simulink model "gm_sampleModel1598_5_sub"  (R2023a)
settings: Solver=VariableStepAuto  StartTime=0.0  StopTime=10.0  RelTol=1e-3
libraries: simulink x3
settings Model: Creator=user1  LastModifiedBy=user1
settings OptimizationCC: BlockReduction=off  ConditionallyExecuteInputs=off
settings DebuggingCC: InheritedTsInSrcMsg=none

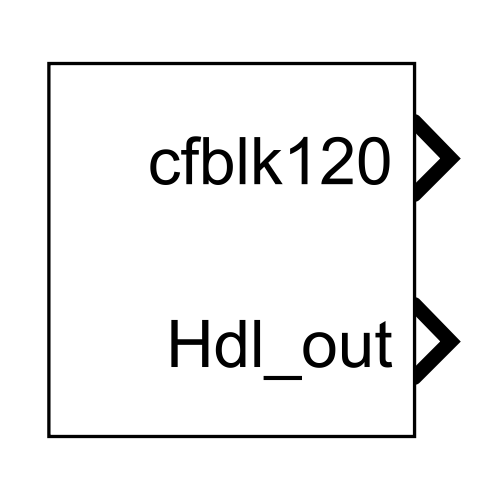
[thumbnail: Simulink's stored preview of the top-level diagram]
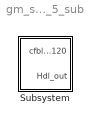
== system gm_sampleModel1598_5_sub ==
  Subsystem : Subsystem

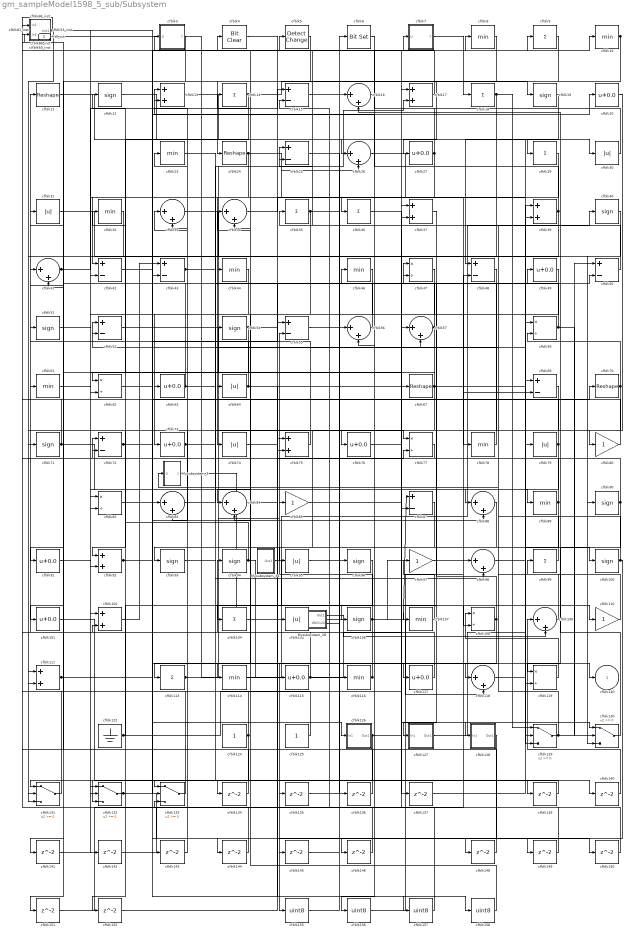
== system gm_sampleModel1598_5_sub/Subsystem ==
  Mysubsystem_28 : Subsystem
  Mysubsystem_3 : Subsystem
  Mysubsystem_34 : Subsystem
  cfblk{8,10,23,32,44,46,61,78,89,107,114,116} (12 alike) : MinMax  OutDataTypeStr=uint8
  cfblk{12,19,40,51,54,71,90,93..94,96,100,106} (12 alike) : Signum
  cfblk{20,27,49,63,73,76,91,101,115,117} (10 alike) : Bias  Bias=0.0  SaturateOnIntegerOverflow=off
  cfblk{13,17,37,39,75,92,102,111} (8 alike) : Sum  OutDataTypeStr=uint8
  cfblk103_inst : Subsystem
  cfblk{9,14,18,29,35..36,99,104,113} (9 alike) : Sum  Inputs=+  OutDataTypeStr=uint8
  cfblk{30..31,64,74,79,95,105} (7 alike) : Abs  OutDataTypeStr=uint8  SaturateOnIntegerOverflow=off
  cfblk{47,59,62,77,82,108,119} (7 alike) : Product  Inputs=*/  OutDataTypeStr=uint8  RndMeth=Zero  SaturateOnIntegerOverflow=on
  cfblk{16,26,33..34,41,56..57,83..84,88,98,109,118} (13 alike) : Sum  Inputs=|++  OutDataTypeStr=uint8
  cfblk{11,24,67,70} (4 alike) : Reshape
  cfblk{80,85,97,110} (4 alike) : Gain  OutDataTypeStr=uint8
  cfblk122 : Ground
  cfblk124 : Constant  OutDataTypeStr=uint8  SampleTime=-1
  cfblk125 : Constant  OutDataTypeStr=uint8  SampleTime=-1
  cfblk126 : Subsystem
  cfblk127 : Subsystem
  cfblk128 : Subsystem
  cfblk{129..133} (5 alike) : Switch  OutDataTypeStr=uint8  SaturateOnIntegerOverflow=off  InputSameDT=off
  cfblk{134..137,139..146,148..152} (17 alike) : Delay  SampleTime=1
  cfblk{15,25,42..43,48,50,52,55,69,72,87} (11 alike) : Sum  Inputs=+-  OutDataTypeStr=uint8
  cfblk{155..158} (4 alike) : DataTypeConversion  OutDataTypeStr=uint8  SaturateOnIntegerOverflow=off  RndMeth=Floor
  cfblk21_inst : Subsystem
  cfblk28_inst : Subsystem
  cfblk3 : Subsystem  mask(Detect Rise Positive){vinit=double(0), InputProcessing=Elements as channels (sample based), OutDataTypeStr=uint8}
      mask prompts: vinit "Simulink:masks:InitialCondition_MP"; InputProcessing "Simulink:masks:InputProcessing_MP"; OutDataTypeStr "Simulink:masks:OutputDataType_MP"
      mask help: Simulink:masks:DetectRisePositive_MD
      mask init:
      | InputProcessing = 'Elements as channels (sample based)';
      | OutDataTypeStr = 'uint8';
      | vinit = double(0);
      mask TypeOptions InputProcessing: Simulink:masks:ColumnsAsChannelsFrameBased | Simulink:masks:ElementsAsChannelsSampleBased
      mask TypeOptions OutDataTypeStr: Simulink:masks:uint8 | Simulink:masks:boolean
      mask Display: fprintf('U > 0\n&  NOT\nU/z > 0')
  cfblk38_inst : Subsystem
  cfblk4 : simulink/Logic and Bit Operations/Bit Clear  iBit=0
      settings: LibrarySourceBlock=|
      | hdlsllib/Logic and Bit
      | Operations/Bit Clear
  cfblk5 : simulink/Logic and Bit Operations/Detect Change  vinit=0  OutDataTypeStr=uint8
      settings: LibrarySourceBlock=|
      | hdlsllib/Logic and Bit
      | Operations/Detect
      | Change
  cfblk53_inst : Subsystem
  cfblk6 : simulink/Logic and Bit Operations/Bit Set  iBit=0
      settings: LibrarySourceBlock=|
      | hdlsllib/Logic and Bit
      | Operations/Bit Set
  cfblk60_inst : Subsystem
  cfblk68_inst : Subsystem
  cfblk7 : Subsystem  mask(Detect Fall Nonpositive){vinit=double(0), InputProcessing=Elements as channels (sample based), OutDataTypeStr=uint8}
      mask prompts: vinit "Simulink:masks:InitialCondition_MP"; InputProcessing "Simulink:masks:InputProcessing_MP"; OutDataTypeStr "Simulink:masks:OutputDataType_MP"
      mask help: Simulink:masks:DetectFallNonpositive_MD
      mask init:
      | InputProcessing = 'Elements as channels (sample based)';
      | OutDataTypeStr = 'uint8';
      | vinit = double(0);
      mask TypeOptions InputProcessing: Simulink:masks:ColumnsAsChannelsFrameBased | Simulink:masks:ElementsAsChannelsSampleBased
      mask TypeOptions OutDataTypeStr: Simulink:masks:uint8 | Simulink:masks:boolean
      mask Display: fprintf('U <= 0\n&  NOT\nU/z <= 0')
  cfblk81_inst : Subsystem
  cfblk86_inst : Subsystem
  cfblk120 : Outport  OutDataTypeStr=uint8  SampleTime=1  VectorParamsAs1DForOutWhenUnconnected=off
  Hdl_out : Outport  Port=2  OutDataTypeStr=uint8  SampleTime=1
  wires:
  Mysubsystem_28/1(Out1) -> cfblk109/2
  Mysubsystem_28/2(cfblk120) -> cfblk120/1
  Mysubsystem_3/1(Out1) -> Mysubsystem_28/1(In1)
  Mysubsystem_34/1(Out1) -> cfblk106/1
  cfblk10/1 -> cfblk56/2, cfblk24/1
  cfblk100/1 -> cfblk148/1, Mysubsystem_3/1(U)
  cfblk101/1 -> cfblk134/1
  cfblk102/1 -> cfblk43/1
  cfblk103_inst/1(out1) -> cfblk38_inst/2(in2)
  cfblk104/1 -> cfblk110/1
  cfblk105/1 -> cfblk98/1
  cfblk106/1 -> cfblk87/1, cfblk55/2, cfblk118/2, cfblk102/2
  cfblk107/1 -> cfblk97/1
  cfblk108/1 -> cfblk155/1, cfblk47/1, cfblk113/1
  cfblk109/1 -> cfblk99/1
  cfblk11/1 -> cfblk29/1
  cfblk110/1 -> cfblk35/1
  cfblk111/1 -> cfblk55/1, cfblk140/1
  cfblk113/1 -> cfblk17/2, cfblk85/1
  cfblk114/1 -> cfblk40/1
  cfblk115/1 -> cfblk87/2, cfblk81_inst/2(in2)
  cfblk116/1 -> cfblk94/1, cfblk11/1, Hdl_out/1
  cfblk117/1 -> cfblk103_inst/1(in1)
  cfblk118/1 -> cfblk79/1
  cfblk119/1 -> cfblk108/1
  cfblk12/1 -> cfblk26/1
  cfblk122/1 -> cfblk57/1, cfblk52/1
  cfblk124/1 -> cfblk53_inst/2(in2), cfblk33/2, cfblk133/1
  cfblk125/1 -> cfblk72/1
  cfblk126/1(Out1) -> cfblk37/1, cfblk132/3
  cfblk127/1(Out1) -> cfblk39/1
  cfblk128/1(Out1) -> cfblk145/1
  cfblk129/1 -> cfblk52/2, cfblk50/1, cfblk61/1
  cfblk13/1 -> cfblk69/1
  cfblk130/1 -> cfblk16/2
  cfblk131/1 -> cfblk60_inst/2(in2)
  cfblk132/1 -> cfblk88/2, cfblk144/1
  cfblk133/1 -> cfblk68_inst/2(in2)
  cfblk134/1 -> cfblk41/1
  cfblk135/1 -> cfblk16/1
  cfblk136/1 -> cfblk68_inst/1(in1)
  cfblk137/1 -> cfblk39/2
  cfblk139/1 -> cfblk131/1
  cfblk14/1 -> cfblk19/1, cfblk62/1
  cfblk140/1 -> cfblk109/1
  cfblk141/1 -> cfblk37/2
  cfblk142/1 -> cfblk48/2
  cfblk143/1 -> cfblk13/1
  cfblk144/1 -> cfblk21_inst/1(in1)
  cfblk145/1 -> cfblk56/1
  cfblk146/1 -> cfblk133/3
  cfblk148/1 -> cfblk86_inst/2(in2)
  cfblk149/1 -> cfblk15/2
  cfblk15/1 -> cfblk9/1
  cfblk150/1 -> cfblk84/2
  cfblk151/1 -> cfblk75/2
  cfblk152/1 -> cfblk67/1
  cfblk155/1 -> cfblk6/1
  cfblk156/1 -> cfblk49/1
  cfblk157/1 -> cfblk4/1
  cfblk158/1 -> cfblk14/1
  cfblk16/1 -> cfblk76/1
  cfblk17/1 -> cfblk3/1(U)
  cfblk18/1 -> cfblk131/2, cfblk129/1
  cfblk19/1 -> cfblk48/1
  cfblk20/1 -> cfblk80/1
  cfblk21_inst/1(out1) -> cfblk132/1
  cfblk23/1 -> cfblk77/1
  cfblk24/1 -> cfblk74/1, cfblk26/2, cfblk129/3
  cfblk25/1 -> cfblk136/1
  cfblk26/1 -> cfblk78/1
  cfblk27/1 -> cfblk38_inst/1(in1), cfblk62/2
  cfblk28_inst/1(out1) -> cfblk30/1, cfblk111/2
  cfblk29/1 -> cfblk42/1
  cfblk3/1(Y) -> cfblk141/1
  cfblk30/1 -> cfblk103_inst/2(in2)
  cfblk31/1 -> cfblk44/1
  cfblk32/1 -> cfblk42/2
  cfblk33/1 -> cfblk90/1
  cfblk34/1 -> cfblk36/1
  cfblk35/1 -> cfblk132/2, cfblk118/1, cfblk5/1
  cfblk36/1 -> cfblk130/1
  cfblk37/1 -> cfblk127/1(In1)
  cfblk38_inst/1(out1) -> cfblk82/1, cfblk150/1
  cfblk39/1 -> cfblk13/2, cfblk101/1
  cfblk4/1 -> cfblk158/1
  cfblk40/1 -> cfblk130/3
  cfblk41/1 -> cfblk15/1, cfblk151/1
  cfblk42/1 -> cfblk8/1
  cfblk43/1 -> cfblk98/2, cfblk108/2
  cfblk44/1 -> cfblk73/1
  cfblk46/1 -> cfblk104/1
  cfblk47/1 -> cfblk146/1
  cfblk48/1 -> cfblk92/1
  cfblk49/1 -> cfblk82/2
  cfblk5/1 -> cfblk43/2
  cfblk50/1 -> cfblk25/1
  cfblk51/1 -> cfblk64/1
  cfblk52/1 -> cfblk137/1
  cfblk53_inst/1(out1) -> cfblk117/1
  cfblk54/1 -> cfblk91/1, cfblk50/2
  cfblk55/1 -> cfblk17/1
  cfblk56/1 -> cfblk33/1
  cfblk57/1 -> cfblk92/2, cfblk21_inst/2(in2)
  cfblk59/1 -> cfblk34/2, cfblk28_inst/2(in2), cfblk130/2
  cfblk6/1 -> cfblk156/1
  cfblk60_inst/1(out1) -> cfblk54/1, cfblk111/1, cfblk139/1
  cfblk61/1 -> cfblk88/1
  cfblk62/1 -> cfblk83/1
  cfblk63/1 -> cfblk28_inst/1(in1), cfblk25/2, cfblk32/1
  cfblk64/1 -> cfblk31/1, cfblk105/1
  cfblk67/1 -> cfblk95/1, cfblk83/2, cfblk63/1, cfblk119/2
  cfblk68_inst/1(out1) -> cfblk71/1, cfblk126/1(In1)
  cfblk69/1 -> cfblk84/1
  cfblk7/1(Y) -> cfblk18/1
  cfblk70/1 -> cfblk131/3, cfblk59/2
  cfblk71/1 -> cfblk53_inst/1(in1), cfblk116/1, cfblk89/1
  cfblk72/1 -> cfblk70/1, cfblk20/1
  cfblk73/1 -> cfblk59/1, cfblk47/2
  cfblk74/1 -> cfblk149/1
  cfblk75/1 -> cfblk41/2
  cfblk76/1 -> cfblk10/1
  cfblk77/1 -> cfblk72/2
  cfblk78/1 -> cfblk46/1
  cfblk79/1 -> cfblk60_inst/1(in1), cfblk129/2
  cfblk8/1 -> cfblk27/1
  cfblk80/1 -> cfblk34/1
  cfblk81_inst/1(out1) -> cfblk102/1
  cfblk82/1 -> cfblk157/1
  cfblk83/1 -> cfblk57/2
  cfblk84/1 -> cfblk77/2
  cfblk85/1 -> cfblk128/1(In1)
  cfblk86_inst/1(out1) -> cfblk81_inst/1(in1)
  cfblk87/1 -> cfblk114/1
  cfblk88/1 -> cfblk93/1
  cfblk89/1 -> cfblk51/1, cfblk107/1
  cfblk9/1 -> cfblk133/2
  cfblk90/1 -> cfblk86_inst/1(in1), cfblk119/1
  cfblk91/1 -> cfblk142/1
  cfblk92/1 -> cfblk143/1, cfblk7/1(U)
  cfblk93/1 -> cfblk135/1
  cfblk94/1 -> cfblk12/1, cfblk115/1, cfblk23/1
  cfblk95/1 -> cfblk96/1
  cfblk96/1 -> cfblk152/1
  cfblk97/1 -> cfblk69/2
  cfblk98/1 -> cfblk100/1
  cfblk99/1 -> cfblk75/1

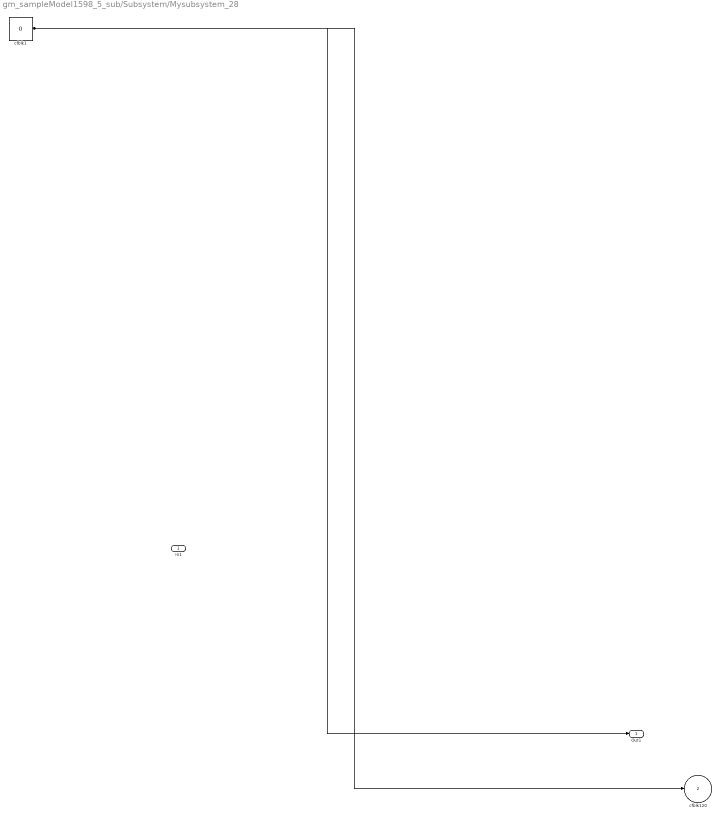
== system gm_sampleModel1598_5_sub/Subsystem/Mysubsystem_28 ==
  In1 : Inport  OutDataTypeStr=uint8  PortDimensions=1  SampleTime=1
  cfblk1 : Constant  Value=0  OutDataTypeStr=uint8  SampleTime=1
  Out1 : Outport  SampleTime=1
  cfblk120 : Outport  Port=2  SampleTime=1  VectorParamsAs1DForOutWhenUnconnected=off
  wires:
  cfblk1/1 -> Out1/1, cfblk120/1

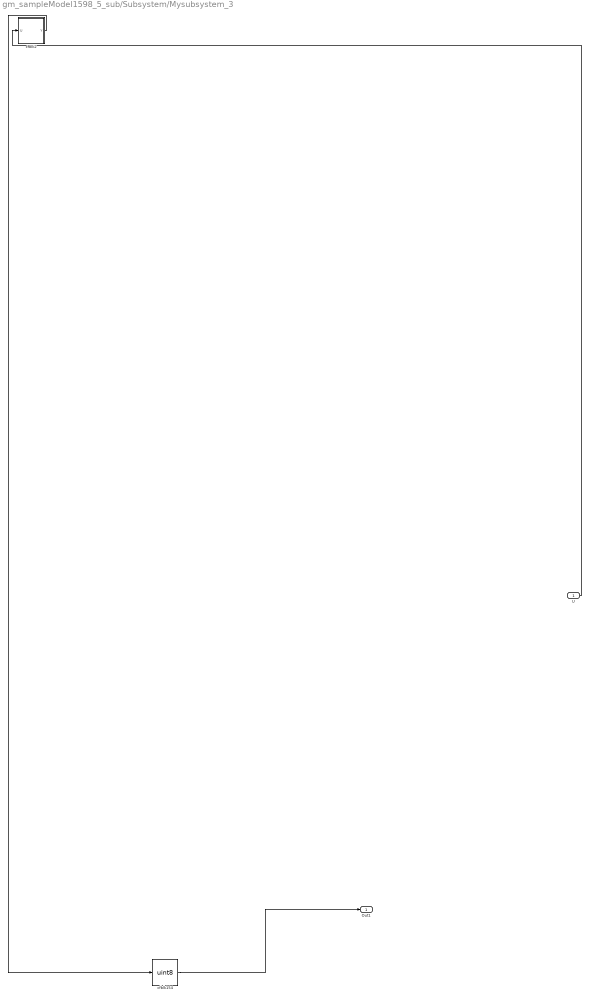
== system gm_sampleModel1598_5_sub/Subsystem/Mysubsystem_3 ==
  U : Inport  OutDataTypeStr=uint8  PortDimensions=1  SampleTime=1
  cfblk154 : DataTypeConversion  OutDataTypeStr=uint8  SaturateOnIntegerOverflow=off  RndMeth=Floor
  cfblk2 : Subsystem  mask(Detect Fall Negative){vinit=double(0), InputProcessing=Elements as channels (sample based), OutDataTypeStr=boolean}
      mask prompts: vinit "Simulink:masks:InitialCondition_MP"; InputProcessing "Simulink:masks:InputProcessing_MP"; OutDataTypeStr "Simulink:masks:OutputDataType_MP"
      mask help: Simulink:masks:DetectFallNegative_MD
      mask init:
      | InputProcessing = 'Elements as channels (sample based)';
      | OutDataTypeStr = 'boolean';
      | vinit = double(0);
      mask TypeOptions InputProcessing: Simulink:masks:ColumnsAsChannelsFrameBased | Simulink:masks:ElementsAsChannelsSampleBased
      mask TypeOptions OutDataTypeStr: Simulink:masks:uint8 | Simulink:masks:boolean
      mask Display: fprintf('U < 0\n&  NOT\nU/z < 0')
  Out1 : Outport  SampleTime=1
  wires:
  U/1 -> cfblk2/1(U)
  cfblk154/1 -> Out1/1
  cfblk2/1(Y) -> cfblk154/1

== system gm_sampleModel1598_5_sub/Subsystem/Mysubsystem_34 ==
  cfblk123 : Subsystem  mask(Counter Limited){uplimit=double(7), tsamp=double(-1)}
      mask prompts: uplimit "Simulink:masks:UpperLimit_MP"; tsamp "Simulink:masks:SampleTime_MP"
      mask help: Simulink:masks:CounterLimited_MD
      mask init:
      | nbits = double(8);
      | tsamp = double(-1);
      | uplimit = double(7);
  cfblk66 : Abs  SaturateOnIntegerOverflow=off
  Out1 : Outport  SampleTime=1
  wires:
  cfblk123/1(y) -> cfblk66/1
  cfblk66/1 -> Out1/1

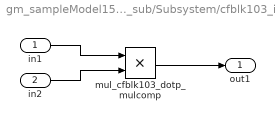
== system gm_sampleModel1598_5_sub/Subsystem/cfblk103_inst ==
  in1 : Inport  OutDataTypeStr=uint8  SampleTime=1
  in2 : Inport  Port=2  OutDataTypeStr=uint8  SampleTime=1
  mul_cfblk103_dotp_mulcomp : Product  Inputs=**  OutDataTypeStr=uint8  SampleTime=1
  out1 : Outport  OutDataTypeStr=uint8  SampleTime=1
  wires:
  in1/1 -> mul_cfblk103_dotp_mulcomp/1
  in2/1 -> mul_cfblk103_dotp_mulcomp/2
  mul_cfblk103_dotp_mulcomp/1 -> out1/1

== system gm_sampleModel1598_5_sub/Subsystem/cfblk126 ==
  In1 : Inport  OutDataTypeStr=uint8  PortDimensions=1  SampleTime=1
  Out1 : Outport  SampleTime=1
  wires:
  In1/1 -> Out1/1

== system gm_sampleModel1598_5_sub/Subsystem/cfblk127 ==
  In1 : Inport  OutDataTypeStr=uint8  PortDimensions=1  SampleTime=1
  Out1 : Outport  SampleTime=1
  wires:
  In1/1 -> Out1/1

== system gm_sampleModel1598_5_sub/Subsystem/cfblk128 ==
  In1 : Inport  OutDataTypeStr=uint8  PortDimensions=1  SampleTime=1
  Out1 : Outport  SampleTime=1
  wires:
  In1/1 -> Out1/1

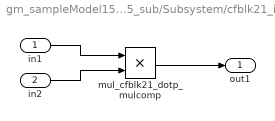
== system gm_sampleModel1598_5_sub/Subsystem/cfblk21_inst ==
  in1 : Inport  OutDataTypeStr=uint8  SampleTime=1
  in2 : Inport  Port=2  OutDataTypeStr=uint8  SampleTime=1
  mul_cfblk21_dotp_mulcomp : Product  Inputs=**  OutDataTypeStr=uint8  SampleTime=1
  out1 : Outport  OutDataTypeStr=uint8  SampleTime=1
  wires:
  in1/1 -> mul_cfblk21_dotp_mulcomp/1
  in2/1 -> mul_cfblk21_dotp_mulcomp/2
  mul_cfblk21_dotp_mulcomp/1 -> out1/1

== system gm_sampleModel1598_5_sub/Subsystem/cfblk28_inst ==
  in1 : Inport  OutDataTypeStr=uint8  SampleTime=1
  in2 : Inport  Port=2  OutDataTypeStr=uint8  SampleTime=1
  mul_cfblk28_dotp_mulcomp : Product  Inputs=**  OutDataTypeStr=uint8  SampleTime=1
  out1 : Outport  OutDataTypeStr=uint8  SampleTime=1
  wires:
  in1/1 -> mul_cfblk28_dotp_mulcomp/1
  in2/1 -> mul_cfblk28_dotp_mulcomp/2
  mul_cfblk28_dotp_mulcomp/1 -> out1/1

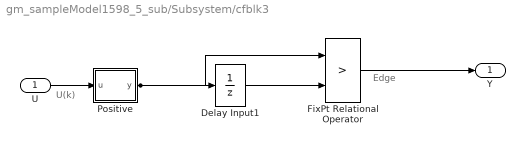
== system gm_sampleModel1598_5_sub/Subsystem/cfblk3 ==
  note: U(k)
  note: Edge
  U : Inport  OutDataTypeStr=uint8  SampleTime=1
  Delay Input1 : UnitDelay  Description=Store in Global RAM  DisableCoverage=on  InitialCondition=vinit  SampleTime=-1  HasFrameUpgradeWarning=on
  FixPt Relational Operator : RelationalOperator  Operator=>  OutDataTypeStr=fixdt(0, 8)  ZeroCross=off  InputSameDT=off
  Positive : Subsystem  mask(Compare To Zero){relop=>, OutDataTypeStr=boolean, ZeroCross=off}
      mask prompts: relop "Simulink:masks:Operator_MP"; OutDataTypeStr "Simulink:masks:OutputDataType_MP"; ZeroCross "Simulink:masks:EnableZerocrossingDetection_MP"
      mask help: Simulink:masks:CompareToZero_MD
      mask init:
      | OutDataTypeStr = 'boolean';
      | ZeroCross = 'off';
      | blkName = 'sampleModel1598_5_sub/Subsystem/cfblk3/Positive';
      | relop = '>';
      | setValue = 'boolean';
      mask TypeOptions relop: == | ~= | < | <= | >= | >
      mask TypeOptions OutDataTypeStr: Simulink:masks:uint8 | Simulink:masks:boolean
      mask Callback ZeroCross: sl('zeroCrossEnable', gcbh);
      mask Display: disp([relop,' 0'])
  Y : Outport  SampleTime=1
  wires:
  U/1 -> Positive/1(u)
  Delay Input1/1 -> FixPt Relational Operator/2
  FixPt Relational Operator/1 -> Y/1
  Positive/1(y) -> FixPt Relational Operator/1, Delay Input1/1

== system gm_sampleModel1598_5_sub/Subsystem/cfblk38_inst ==
  in1 : Inport  OutDataTypeStr=uint8  SampleTime=1
  in2 : Inport  Port=2  OutDataTypeStr=uint8  SampleTime=1
  mul_cfblk38_dotp_mulcomp : Product  Inputs=**  OutDataTypeStr=uint8  SampleTime=1
  out1 : Outport  OutDataTypeStr=uint8  SampleTime=1
  wires:
  in1/1 -> mul_cfblk38_dotp_mulcomp/1
  in2/1 -> mul_cfblk38_dotp_mulcomp/2
  mul_cfblk38_dotp_mulcomp/1 -> out1/1

== system gm_sampleModel1598_5_sub/Subsystem/cfblk53_inst ==
  in1 : Inport  OutDataTypeStr=uint8  SampleTime=1
  in2 : Inport  Port=2  OutDataTypeStr=uint8  SampleTime=1
  mul_cfblk53_dotp_mulcomp : Product  Inputs=**  OutDataTypeStr=uint8  SampleTime=1
  out1 : Outport  OutDataTypeStr=uint8  SampleTime=1
  wires:
  in1/1 -> mul_cfblk53_dotp_mulcomp/1
  in2/1 -> mul_cfblk53_dotp_mulcomp/2
  mul_cfblk53_dotp_mulcomp/1 -> out1/1

== system gm_sampleModel1598_5_sub/Subsystem/cfblk60_inst ==
  in1 : Inport  OutDataTypeStr=uint8  SampleTime=1
  in2 : Inport  Port=2  OutDataTypeStr=uint8  SampleTime=1
  mul_cfblk60_dotp_mulcomp : Product  Inputs=**  OutDataTypeStr=uint8  SampleTime=1
  out1 : Outport  OutDataTypeStr=uint8  SampleTime=1
  wires:
  in1/1 -> mul_cfblk60_dotp_mulcomp/1
  in2/1 -> mul_cfblk60_dotp_mulcomp/2
  mul_cfblk60_dotp_mulcomp/1 -> out1/1

== system gm_sampleModel1598_5_sub/Subsystem/cfblk68_inst ==
  in1 : Inport  OutDataTypeStr=uint8  SampleTime=1
  in2 : Inport  Port=2  OutDataTypeStr=uint8  SampleTime=1
  mul_cfblk68_dotp_mulcomp : Product  Inputs=**  OutDataTypeStr=uint8  SampleTime=1
  out1 : Outport  OutDataTypeStr=uint8  SampleTime=1
  wires:
  in1/1 -> mul_cfblk68_dotp_mulcomp/1
  in2/1 -> mul_cfblk68_dotp_mulcomp/2
  mul_cfblk68_dotp_mulcomp/1 -> out1/1

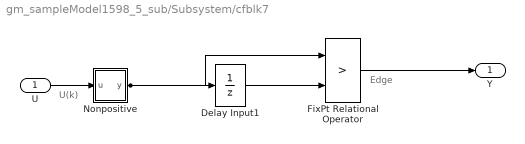
== system gm_sampleModel1598_5_sub/Subsystem/cfblk7 ==
  note: U(k)
  note: Edge
  U : Inport  OutDataTypeStr=uint8  SampleTime=1
  Delay Input1 : UnitDelay  Description=Store in Global RAM  DisableCoverage=on  InitialCondition=vinit  SampleTime=-1  HasFrameUpgradeWarning=on
  FixPt Relational Operator : RelationalOperator  Operator=>  OutDataTypeStr=fixdt(0, 8)  ZeroCross=off  InputSameDT=off
  Nonpositive : Subsystem  mask(Compare To Zero){relop=<=, OutDataTypeStr=boolean, ZeroCross=off}
      mask prompts: relop "Simulink:masks:Operator_MP"; OutDataTypeStr "Simulink:masks:OutputDataType_MP"; ZeroCross "Simulink:masks:EnableZerocrossingDetection_MP"
      mask help: Simulink:masks:CompareToZero_MD
      mask init:
      | OutDataTypeStr = 'boolean';
      | ZeroCross = 'off';
      | blkName = 'sampleModel1598_5_sub/Subsystem/cfblk7/Nonpositive';
      | relop = '<=';
      | setValue = 'boolean';
      mask TypeOptions relop: == | ~= | < | <= | >= | >
      mask TypeOptions OutDataTypeStr: Simulink:masks:uint8 | Simulink:masks:boolean
      mask Callback ZeroCross: sl('zeroCrossEnable', gcbh);
      mask Display: disp([relop,' 0'])
  Y : Outport  SampleTime=1
  wires:
  U/1 -> Nonpositive/1(u)
  Delay Input1/1 -> FixPt Relational Operator/2
  FixPt Relational Operator/1 -> Y/1
  Nonpositive/1(y) -> FixPt Relational Operator/1, Delay Input1/1

== system gm_sampleModel1598_5_sub/Subsystem/cfblk81_inst ==
  in1 : Inport  OutDataTypeStr=uint8  SampleTime=1
  in2 : Inport  Port=2  OutDataTypeStr=uint8  SampleTime=1
  mul_cfblk81_dotp_mulcomp : Product  Inputs=**  OutDataTypeStr=uint8  SampleTime=1
  out1 : Outport  OutDataTypeStr=uint8  SampleTime=1
  wires:
  in1/1 -> mul_cfblk81_dotp_mulcomp/1
  in2/1 -> mul_cfblk81_dotp_mulcomp/2
  mul_cfblk81_dotp_mulcomp/1 -> out1/1

== system gm_sampleModel1598_5_sub/Subsystem/cfblk86_inst ==
  in1 : Inport  OutDataTypeStr=uint8  SampleTime=1
  in2 : Inport  Port=2  OutDataTypeStr=uint8  SampleTime=1
  mul_cfblk86_dotp_mulcomp : Product  Inputs=**  OutDataTypeStr=uint8  SampleTime=1
  out1 : Outport  OutDataTypeStr=uint8  SampleTime=1
  wires:
  in1/1 -> mul_cfblk86_dotp_mulcomp/1
  in2/1 -> mul_cfblk86_dotp_mulcomp/2
  mul_cfblk86_dotp_mulcomp/1 -> out1/1

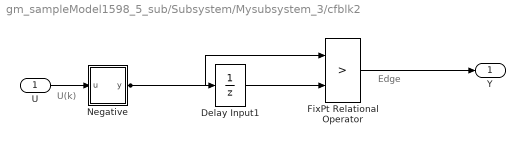
== system gm_sampleModel1598_5_sub/Subsystem/Mysubsystem_3/cfblk2 ==
  note: U(k)
  note: Edge
  U : Inport  OutDataTypeStr=uint8  SampleTime=1
  Delay Input1 : UnitDelay  Description=Store in Global RAM  DisableCoverage=on  InitialCondition=vinit  SampleTime=-1  HasFrameUpgradeWarning=on
  FixPt Relational Operator : RelationalOperator  Operator=>  OutDataTypeStr=boolean  ZeroCross=off  InputSameDT=off
  Negative : Subsystem  mask(Compare To Zero){relop=<, OutDataTypeStr=boolean, ZeroCross=off}
      mask prompts: relop "Simulink:masks:Operator_MP"; OutDataTypeStr "Simulink:masks:OutputDataType_MP"; ZeroCross "Simulink:masks:EnableZerocrossingDetection_MP"
      mask help: Simulink:masks:CompareToZero_MD
      mask init:
      | OutDataTypeStr = 'boolean';
      | ZeroCross = 'off';
      | blkName = 'sampleModel1598_5_sub/Subsystem/Mysubsystem_3/cfblk2/Negative';
      | relop = '<';
      | setValue = 'boolean';
      mask TypeOptions relop: == | ~= | < | <= | >= | >
      mask TypeOptions OutDataTypeStr: Simulink:masks:uint8 | Simulink:masks:boolean
      mask Callback ZeroCross: sl('zeroCrossEnable', gcbh);
      mask Display: disp([relop,' 0'])
  Y : Outport  SampleTime=1
  wires:
  U/1 -> Negative/1(u)
  Delay Input1/1 -> FixPt Relational Operator/2
  FixPt Relational Operator/1 -> Y/1
  Negative/1(y) -> FixPt Relational Operator/1, Delay Input1/1

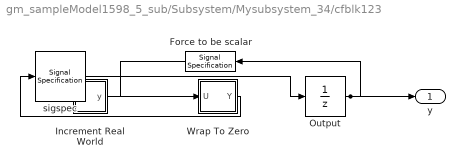
== system gm_sampleModel1598_5_sub/Subsystem/Mysubsystem_34/cfblk123 ==
  Force to be scalar : SignalSpecification  DisableCoverage=on  Dimensions=1
  Increment Real World : Subsystem  mask(Real World Value Increment){}
      mask help: Simulink:masks:RealWorldValueIncrement_MD
      mask Display: disp('V++')
  Output : UnitDelay  InitialCondition=0.0  SampleTime=tsamp  HasFrameUpgradeWarning=on
  Wrap To Zero : Subsystem  mask(Wrap To Zero){Threshold=double(7)}
      mask prompts: Threshold "Simulink:masks:Threshold_MP"
      mask help: Simulink:masks:WrapToZero_MD
  sigspec : SignalSpecification  OutDataTypeStr=uint8  Dimensions=1
  y : Outport  SampleTime=1
  wires:
  Force to be scalar/1 -> Increment Real World/1(u)
  Increment Real World/1(y) -> Wrap To Zero/1(U)
  Output/1 -> Force to be scalar/1, y/1
  Wrap To Zero/1(Y) -> sigspec/1
  sigspec/1 -> Output/1

== system gm_sampleModel1598_5_sub/Subsystem/cfblk3/Positive ==
  u : Inport  OutDataTypeStr=uint8  SampleTime=1
  Compare : RelationalOperator  Operator=>  OutDataTypeStr=boolean  ZeroCross=off
  Constant : Constant  DisableCoverage=on  Value=0  OutDataTypeStr=Inherit: Inherit via back propagation  SampleTime=-1  PreserveConstantTs=on
  y : Outport  SampleTime=1
  wires:
  u/1 -> Compare/1
  Compare/1 -> y/1
  Constant/1 -> Compare/2

== system gm_sampleModel1598_5_sub/Subsystem/cfblk7/Nonpositive ==
  u : Inport  OutDataTypeStr=uint8  SampleTime=1
  Compare : RelationalOperator  Operator=<=  OutDataTypeStr=boolean  ZeroCross=off
  Constant : Constant  DisableCoverage=on  Value=0  OutDataTypeStr=Inherit: Inherit via back propagation  SampleTime=-1  PreserveConstantTs=on
  y : Outport  SampleTime=1
  wires:
  u/1 -> Compare/1
  Compare/1 -> y/1
  Constant/1 -> Compare/2

== system gm_sampleModel1598_5_sub/Subsystem/Mysubsystem_3/cfblk2/Negative ==
  u : Inport  OutDataTypeStr=uint8  SampleTime=1
  Compare : RelationalOperator  Operator=<  OutDataTypeStr=boolean  ZeroCross=off
  Constant : Constant  DisableCoverage=on  Value=0  OutDataTypeStr=Inherit: Inherit via back propagation  SampleTime=-1  PreserveConstantTs=on
  y : Outport  SampleTime=1
  wires:
  u/1 -> Compare/1
  Compare/1 -> y/1
  Constant/1 -> Compare/2

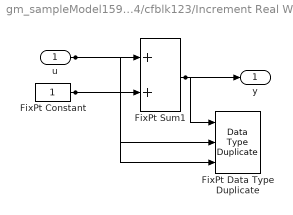
== system gm_sampleModel1598_5_sub/Subsystem/Mysubsystem_34/cfblk123/Increment Real World ==
  u : Inport  OutDataTypeStr=uint8  SampleTime=1
  FixPt Constant : Constant  DisableCoverage=on  OutDataTypeStr=Inherit: Inherit via back propagation  SampleTime=-1
  FixPt Data Type Duplicate : DataTypeDuplicate  DisableCoverage=on  NumInputPorts=3
  FixPt Sum1 : Sum  InputSameDT=on  OutDataTypeStr=Inherit: Inherit via back propagation  LockScale=on
  y : Outport  SampleTime=1
  wires:
  u/1 -> FixPt Sum1/1, FixPt Data Type Duplicate/2
  FixPt Constant/1 -> FixPt Sum1/2, FixPt Data Type Duplicate/3
  FixPt Sum1/1 -> FixPt Data Type Duplicate/1, y/1

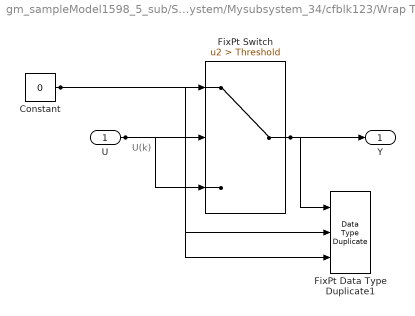
== system gm_sampleModel1598_5_sub/Subsystem/Mysubsystem_34/cfblk123/Wrap To Zero ==
  note: U(k)
  U : Inport  OutDataTypeStr=uint8  SampleTime=1
  Constant : Constant  DisableCoverage=on  Value=0  OutDataTypeStr=Inherit: Inherit via back propagation  SampleTime=-1
  FixPt Data Type Duplicate1 : DataTypeDuplicate  DisableCoverage=on  NumInputPorts=3
  FixPt Switch : Switch  Criteria=u2 > Threshold  Threshold=Threshold  OutDataTypeStr=Inherit: Inherit via back propagation  ZeroCross=off  SaturateOnIntegerOverflow=off  InputSameDT=off
  Y : Outport  SampleTime=1
  wires:
  U/1 -> FixPt Switch/3, FixPt Switch/2, FixPt Data Type Duplicate1/2
  Constant/1 -> FixPt Switch/1, FixPt Data Type Duplicate1/3
  FixPt Switch/1 -> FixPt Data Type Duplicate1/1, Y/1
